simulink model "scheme1"  (R2024a)
settings: Solver=VariableStepAuto  StartTime=0.0  StopTime=10.0  RelTol=1e-8
undefined symbols (not defined in the file): a0, a1, c1, c2, dy0, func, lambda1, lambda2, y0
settings Model: Creator=alexivanov  LastModifiedBy=alexivanov

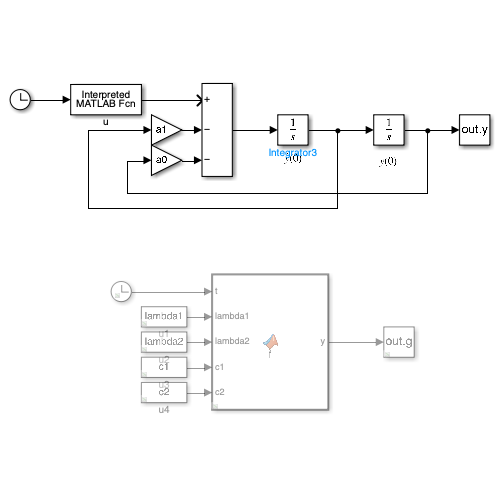
[thumbnail: Simulink's stored preview of the top-level diagram]
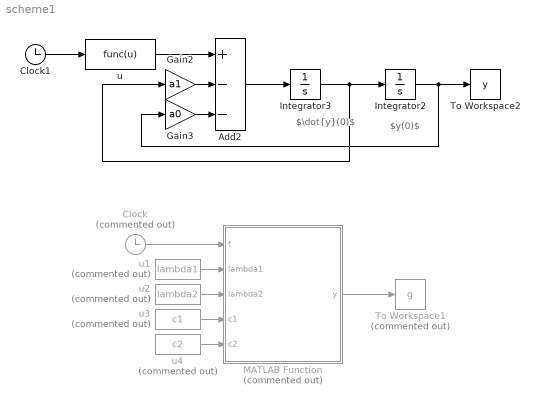
== system scheme1 ==
  note: $\dot{y}(0)$
  note: $y(0)$
  Add2 : Sum  Inputs=+--
  Clock : Clock  Commented=on
  Clock1 : Clock
  Gain2 : Gain  Gain=a1
  Gain3 : Gain  Gain=a0
  Integrator2 : Integrator  InitialCondition=y0
  Integrator3 : Integrator  InitialCondition=dy0
  MATLAB Function : MATLAB Function  Commented=on  TreatAsAtomicUnit=on
  To Workspace1 : ToWorkspace  Commented=on  VariableName=g  SaveFormat=Timeseries  SampleTime=-1
  To Workspace2 : ToWorkspace  VariableName=y  SaveFormat=Timeseries  SampleTime=-1
  u : MATLABFcn  MATLABFcn=func(u)
  u1 : Constant  Commented=on  Value=lambda1  SampleTime=0
  u2 : Constant  Commented=on  Value=lambda2  SampleTime=0
  u3 : Constant  Commented=on  Value=c1  SampleTime=0
  u4 : Constant  Commented=on  Value=c2  SampleTime=0
  wires:
  Clock/1 -> MATLAB Function/1(t)
  MATLAB Function/1(y) -> To Workspace1/1
  u1/1 -> MATLAB Function/2(lambda1)
  Integrator3/1 -> Gain2/1, Integrator2/1
  Add2/1 -> Integrator3/1
  u/1 -> Add2/1
  Gain2/1 -> Add2/2
  Gain3/1 -> Add2/3
  u2/1 -> MATLAB Function/3(lambda2)
  u3/1 -> MATLAB Function/4(c1)
  u4/1 -> MATLAB Function/5(c2)
  Integrator2/1 -> Gain3/1, To Workspace2/1
  Clock1/1 -> u/1

== matlab function scheme1/MATLAB Function ==
  data: t input; y output; lambda1 input; lambda2 input; c1 input; c2 input
function y = f(t, lambda1, lambda2, c1, c2)
    if imag(lambda1) == 0 && imag(lambda2) == 0 && lambda1 ~= lambda2
        y = c1 * exp(lambda1 * t) + c2 * exp(lambda2 * t);
    elseif lambda1 == lambda2
        y = c1 * exp(lambda1 * t) + c2 .* t * exp(lambda2 * t)
    else
        alpha = real(lambda1);
        beta = imag(lambda1);
        y = exp(alpha * t) * (c1 * cos(beta * t) + c2 * sin(beta * t));
    end
